simulink model "parity"  (R2021b)
settings: Solver=VariableStepAuto  StartTime=0.0  StopTime=10.0  RelTol=1e-3
undefined symbols (not defined in the file): Ad, Bdd, Cd, Ddd, gain, Hus, s, sigma_ay, sigma_r, vs
libraries: simulink x5
settings Model: Creator=Sazgar  LastModifiedBy=Sazgar

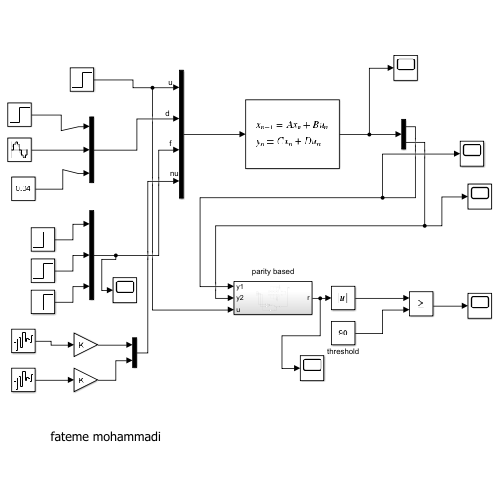
[thumbnail: Simulink's stored preview of the top-level diagram]
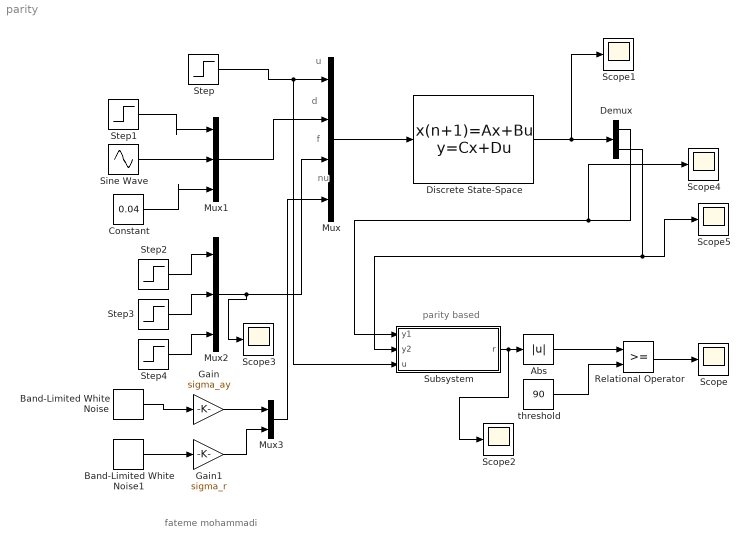
== system parity ==
  note: fateme mohammadi
  note: parity based
  note: nu
  note: f
  note: d
  note: u
  Abs : Abs
  Band-Limited White Noise : simulink/Sources/Band-Limited White Noise  Cov=[1]  Ts=0.01  seed=[1234]
  Band-Limited White Noise1 : simulink/Sources/Band-Limited White Noise  Cov=[1]  Ts=0.01  seed=[5678]
  Constant : Constant  Value=0.04  SampleTime=0.01
  Demux : Demux  Outputs=2
  Discrete State-Space : DiscreteStateSpace  A=Ad  B=Bdd  C=Cd  D=Ddd  SampleTime=0.01
  Gain : Gain  Gain=sigma_ay
  Gain1 : Gain  Gain=sigma_r
  Mux : Mux
  Mux1 : Mux  Inputs=3
  Mux2 : Mux  Inputs=3
  Mux3 : Mux  Inputs=2
  Relational Operator : RelationalOperator  OutDataTypeStr=boolean  RndMeth=Simplest
  Scope{,1..5} (6 alike) : Scope
  Sine Wave : Sin  Amplitude=0.03  Frequency=0.5  SampleTime=0.01
  Step : Step  SampleTime=0.01
  Step1 : Step  Time=3  After=0.05  SampleTime=0.01
  Step2 : Step  Time=3  After=0.5  SampleTime=0.01
  Step3 : Step  Time=5  SampleTime=0.01
  Step4 : Step  Time=7  After=0.8  SampleTime=0.01
  Subsystem : Subsystem
  threshold : Constant  Value=90
  wires:
  Mux/1 -> Discrete State-Space/1
  Step/1 -> Subsystem/3(u), Mux/1
  Step1/1 -> Mux1/1
  Sine Wave/1 -> Mux1/2
  Constant/1 -> Mux1/3
  Mux1/1 -> Mux/2
  Step2/1 -> Mux2/1
  Step3/1 -> Mux2/2
  Step4/1 -> Mux2/3
  Mux2/1 -> Scope3/1, Mux/3
  Band-Limited White Noise1/1 -> Gain1/1
  Band-Limited White Noise/1 -> Gain/1
  Gain/1 -> Mux3/1
  Gain1/1 -> Mux3/2
  Mux3/1 -> Mux/4
  Discrete State-Space/1 -> Demux/1, Scope1/1
  Subsystem/1(r) -> Scope2/1, Abs/1
  Abs/1 -> Relational Operator/1
  threshold/1 -> Relational Operator/2
  Relational Operator/1 -> Scope/1
  Demux/2 -> Subsystem/2(y2), Scope5/1
  Demux/1 -> Subsystem/1(y1), Scope4/1

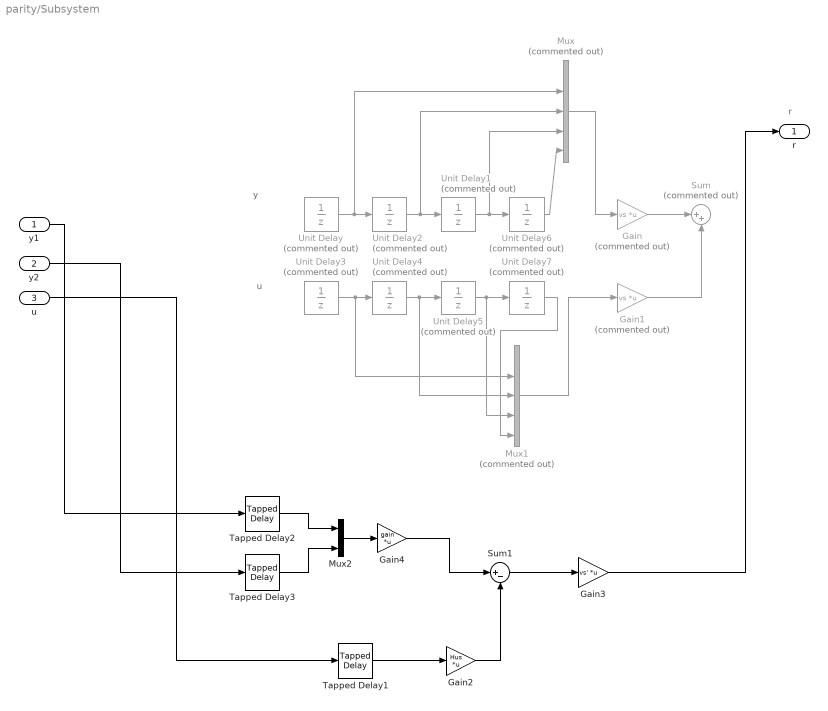
== system parity/Subsystem ==
  note: r
  note: u
  note: y
  y1 : Inport
  y2 : Inport  Port=2
  u : Inport  Port=3
  Gain : Gain  Commented=on  Gain=vs  Multiplication=Matrix(K*u)
  Gain1 : Gain  Commented=on  Gain=vs  Multiplication=Matrix(K*u)
  Gain2 : Gain  Gain=Hus  Multiplication=Matrix(K*u)
  Gain3 : Gain  Gain=vs'  Multiplication=Matrix(K*u)
  Gain4 : Gain  Gain=gain  Multiplication=Matrix(K*u)
  Mux : Mux  Commented=on  Inputs=5
  Mux1 : Mux  Commented=on  Inputs=5
  Mux2 : Mux  Inputs=2
  Sum : Sum  Commented=on  Inputs=|++
  Sum1 : Sum  Inputs=|+-
  Tapped Delay1 : simulink/Discrete/Tapped Delay  vinit=0.0  samptime=0.01  NumDelays=s  DelayOrder=Oldest  includeCurrent=on
  Tapped Delay2 : simulink/Discrete/Tapped Delay  vinit=0.0  samptime=0.01  NumDelays=s  DelayOrder=Oldest  includeCurrent=on
  Tapped Delay3 : simulink/Discrete/Tapped Delay  vinit=0.0  samptime=0.01  NumDelays=s  DelayOrder=Oldest  includeCurrent=on
  Unit Delay{,1..7} (8 alike) : UnitDelay  Commented=on  SampleTime=0.01  HasFrameUpgradeWarning=on
  r : Outport
  wires:
  Unit Delay2/1 -> Mux/3, Unit Delay1/1
  Unit Delay/1 -> Mux/2, Unit Delay2/1
  Unit Delay1/1 -> Unit Delay6/1, Mux/4
  Unit Delay3/1 -> Mux1/2, Unit Delay4/1
  Unit Delay4/1 -> Mux1/3, Unit Delay5/1
  Mux/1 -> Gain/1
  Mux1/1 -> Gain1/1
  Gain/1 -> Sum/1
  Gain1/1 -> Sum/2
  Unit Delay6/1 -> Mux/5
  Unit Delay5/1 -> Mux1/4, Unit Delay7/1
  Unit Delay7/1 -> Mux1/5
  u/1 -> Tapped Delay1/1
  Tapped Delay1/1 -> Gain2/1
  Gain2/1 -> Sum1/2
  Sum1/1 -> Gain3/1
  Gain3/1 -> r/1
  y1/1 -> Tapped Delay2/1
  y2/1 -> Tapped Delay3/1
  Tapped Delay2/1 -> Mux2/1
  Tapped Delay3/1 -> Mux2/2
  Gain4/1 -> Sum1/1
  Mux2/1 -> Gain4/1
